simulink subsystem "massBalances"  (R2024a)
settings: Solver=VariableStepAuto  StartTime=0.0  StopTime=10.0  RelTol=1e-3
settings Model: DefaultTestHarness=massBalances_Harness1  Creator=ilan.malkin  LastModifiedBy=eunice.duplessis

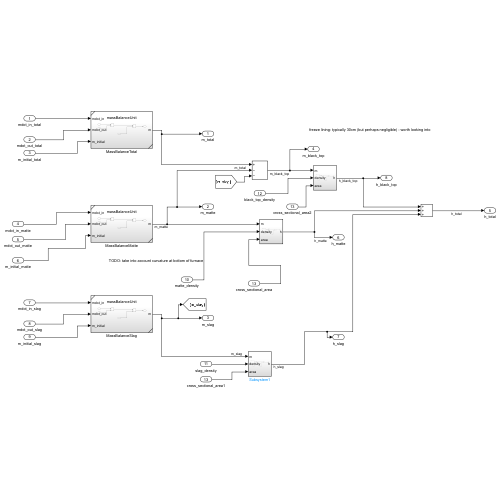
[thumbnail: Simulink's stored preview of the top-level diagram]
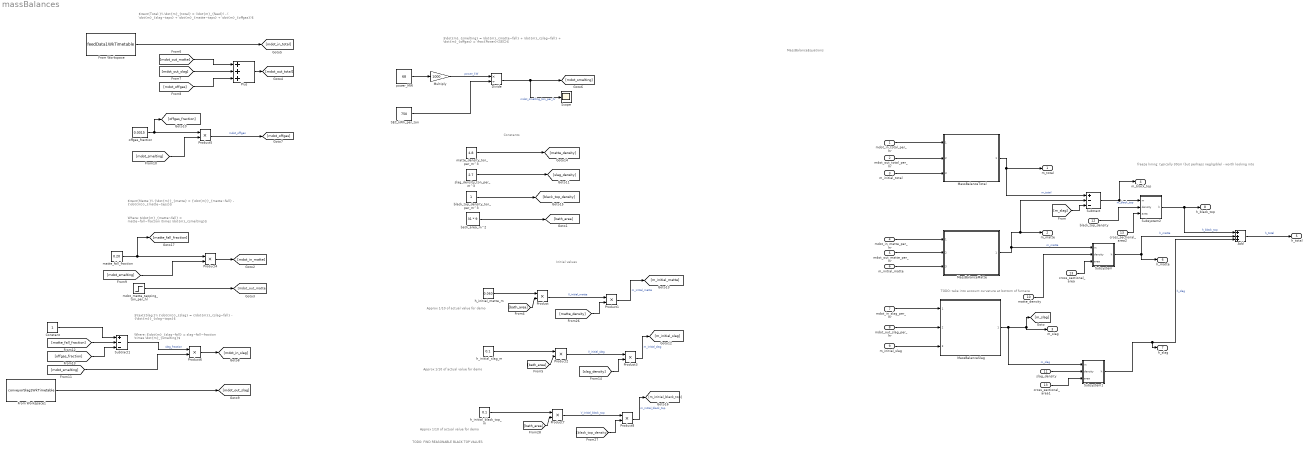
== system massBalances ==
  note: MassBalanceEquations
  note: freeze lining: typically 30cm (but perhaps negligible) - worth looking into
  note: TODO: take into account curvature at bottom of furnace
  note: $\text{Total:}\\ \dot{m}_{total} = (\dot{m}_{feed}) - ( \dot{m}_{slag~taps} + \dot{m}_{matte~taps} + \dot{m}_{offgas})$
  note: Approx 1/10 of actual value for demo
  note: $\text{Matte:}\\ {\dot{m}}_{matte} = {\dot{m}}_{matte~fall} - {\dot{m}}_{matte~taps}$
  note: Constants
  note: Initial values
  note: Approx 1/10 of actual value for demo
  note: Approx 1/10 of actual value for demo
  note: TODO: FIND REASONABLE BLACK TOP VALUES
  note: Where: $\dot{m}_{matte~fall} = matte~fall~fraction \times \dot{m}_{smelting}$
  note: Where: $\dot{m}_{slag~fall} = slag~fall~fraction \times \dot{m}_{smelting}$
  note: $\text{Slag:}\\ {\dot{m}}_{slag} = {\dot{m}}_{slag~fall} - {\dot{m}}_{slag~taps}$
  note: $\dot{m}_{smelting} = \dot{m}_{matte~fall} + \dot{m}_{slag~fall} + \dot{m}_{offgas} = \frac{Power}{SEC}$
  mdot_in_total_per_hr : Inport
  mdot_out_total_per_hr : Inport  Port=2
  m_initial_total : Inport  Port=3
  mdot_in_matte_per_hr : Inport  Port=4
  mdot_out_matte_per_hr : Inport  Port=5
  m_initial_matte : Inport  Port=6
  mdot_in_slag_per_hr : Inport  Port=7
  mdot_out_slag_per_hr : Inport  Port=8
  m_initial_slag : Inport  Port=9
  matte_density : Inport  Port=10
  slag_density : Inport  Port=11
  black_top_density : Inport  Port=12
  cross_sectional_area : Inport  Port=13
  Add : Sum  Inputs=+++
  Constant : Constant
  Divide : Product  Inputs=*/
  From Workspace : FromWorkspace  VariableName=feedData1WkTimetable
  From Workspace1 : FromWorkspace  VariableName=conveyorSlag1WkTimetable
  MassBalanceMatte : Subsystem  ReferencedSubsystem=massBalanceUnit
  MassBalanceSlag : Subsystem  ReferencedSubsystem=massBalanceUnit
  MassBalanceTotal : Subsystem  ReferencedSubsystem=massBalanceUnit
  Multiply : Gain  Gain=1000
  Plus : Sum  Inputs=+++
  Product{,1..8} (9 alike) : Product
  SEC_kWh_per_ton : Constant  Value=750
  Scope : Scope
  Subsystem : Subsystem
  Subsystem1 : Subsystem
  Subsystem2 : Subsystem
  Subtract : Sum  Inputs=+--
  Subtract1 : Sum  Inputs=+--
  bath_area_m^2 : Constant  Value=31 * 9
  black_top_density_ton_per_m^3 : Constant
  cross_sectional_area1 : InportShadow  Port=13
  cross_sectional_area2 : InportShadow  Port=13
  h_initial_black_top_m : Constant  Value=0.1
  h_initial_matte_m : Constant  Value=0.060
  h_initial_slag_m : Constant  Value=0.1
  matte_density_ton_per_m^3 : Constant  Value=4.8
  matte_fall_fraction : Constant  Value=0.20
  mdot_matte_tapping_ton_per_hr : Step  Time=44  After=1.5  SampleTime=0
  offgas_fraction : Constant  Value=0.0015
  power_MW : Constant  Value=68
  slag_density_ton_per_m^3 : Constant  Value=2.7
  m_total : Outport
  m_matte : Outport  Port=2
  m_slag : Outport  Port=3
  m_black_top : Outport  Port=4
  h_total : Outport  Port=5
  h_matte : Outport  Port=6
  h_slag : Outport  Port=7
  h_black_top : Outport  Port=8
  wires:
  MassBalanceMatte/1 -> Subsystem/1(m), Subtract/2, m_matte/1  "m_matte"
  mdot_in_matte_per_hr/1 -> MassBalanceMatte/1
  mdot_out_matte_per_hr/1 -> MassBalanceMatte/2
  m_initial_matte/1 -> MassBalanceMatte/3
  mdot_in_total_per_hr/1 -> MassBalanceTotal/1
  mdot_out_total_per_hr/1 -> MassBalanceTotal/2
  m_initial_total/1 -> MassBalanceTotal/3
  MassBalanceTotal/1 -> Subtract/1, m_total/1  "m_total"
  matte_density/1 -> Subsystem/2(density)
  cross_sectional_area/1 -> Subsystem/3(area)
  Subsystem/1(h) -> h_matte/1, Add/2  "h_matte"
  slag_density/1 -> Subsystem1/2(density)
  cross_sectional_area1/1 -> Subsystem1/3(area)
  Subsystem1/1(h) -> Add/3, h_slag/1  "h_slag"
  Add/1 -> h_total/1  "h_total"
  MassBalanceSlag/1 -> [m_slag], m_slag/1, Subsystem1/1(m)  "m_slag"
  m_initial_slag/1 -> MassBalanceSlag/3
  mdot_out_slag_per_hr/1 -> MassBalanceSlag/2
  mdot_in_slag_per_hr/1 -> MassBalanceSlag/1
  [m_slag] -> Subtract/3
  Subtract/1 -> m_black_top/1, Subsystem2/1(m)  "m_black_top"
  cross_sectional_area2/1 -> Subsystem2/3(area)
  black_top_density/1 -> Subsystem2/2(density)
  Subsystem2/1(h) -> Add/1, h_black_top/1  "h_black_top"
  mdot_matte_tapping_ton_per_hr/1 -> [mdot_out_matte]
  Product/1 -> Product1/1  "V_initial_matte"
  slag_density_ton_per_m^3/1 -> [slag_density]
  Product1/1 -> [m_initial_matte]  "m_initial_matte"
  [black_top_density] -> Product8/2
  Product7/1 -> Product8/1  "V_initial_black_top"
  Product2/1 -> Product3/1  "V_initial_slag"
  Multiply/1 -> Divide/1  "power_kW"
  offgas_fraction/1 -> Product5/1, [offgas_fraction]
  matte_fall_fraction/1 -> Product4/1, [matte_fall_fraction]
  [bath_area] -> Product2/2
  Constant/1 -> Subtract1/1
  SEC_kWh_per_ton/1 -> Divide/2
  [mdot_out_matte] -> Plus/1
  [mdot_offgas] -> Plus/3
  Subtract1/1 -> Product6/1  "slag_fraction"
  Product6/1 -> [mdot_in_slag]
  [bath_area] -> Product/2
  Product3/1 -> [m_initial_slag]  "m_initial_slag"
  [offgas_fraction] -> Subtract1/3
  matte_density_ton_per_m^3/1 -> [matte_density]
  Divide/1 -> [mdot_smelting], Scope/1  "mdot_smelting_ton_per_hr"
  Plus/1 -> [mdot_out_total]
  [mdot_smelting] -> Product6/2
  [mdot_smelting] -> Product5/2
  power_MW/1 -> Multiply/1
  black_top_density_ton_per_m^3/1 -> [black_top_density]
  [slag_density] -> Product3/2
  From Workspace/1 -> [mdot_in_total]
  [matte_fall_fraction] -> Subtract1/2
  h_initial_matte_m/1 -> Product/1
  From Workspace1/1 -> [mdot_out_slag]
  [mdot_out_slag] -> Plus/2
  Product8/1 -> [m_initial_black_top]  "m_initial_black_top"
  bath_area_m^2/1 -> [bath_area]
  [bath_area] -> Product7/2
  Product4/1 -> [mdot_in_matte]
  Product5/1 -> [mdot_offgas]  "mdot_offgas"
  h_initial_black_top_m/1 -> Product7/1
  [matte_density] -> Product1/2
  [mdot_smelting] -> Product4/2
  h_initial_slag_m/1 -> Product2/1

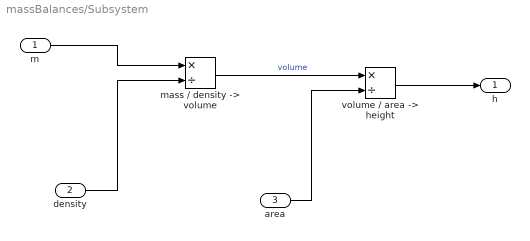
== system massBalances/Subsystem ==
  m : Inport
  density : Inport  Port=2
  area : Inport  Port=3
  "mass / density -> volume" : Product  Inputs=*/
  "volume / area -> height" : Product  Inputs=*/
  h : Outport
  wires:
  "mass / density -> volume"/1 -> "volume / area -> height"/1  "volume"
  density/1 -> "mass / density -> volume"/2
  "volume / area -> height"/1 -> h/1
  m/1 -> "mass / density -> volume"/1
  area/1 -> "volume / area -> height"/2

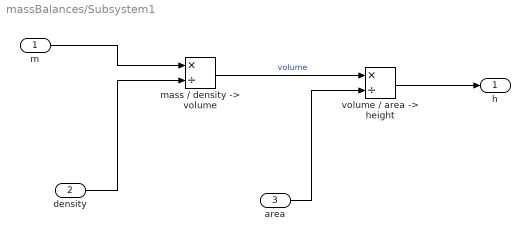
== system massBalances/Subsystem1 ==
  m : Inport
  density : Inport  Port=2
  area : Inport  Port=3
  "mass / density -> volume" : Product  Inputs=*/
  "volume / area -> height" : Product  Inputs=*/
  h : Outport
  wires:
  area/1 -> "volume / area -> height"/2
  m/1 -> "mass / density -> volume"/1
  "volume / area -> height"/1 -> h/1
  density/1 -> "mass / density -> volume"/2
  "mass / density -> volume"/1 -> "volume / area -> height"/1  "volume"

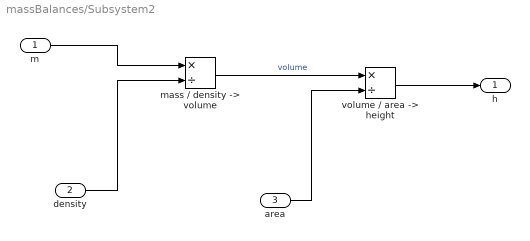
== system massBalances/Subsystem2 ==
  m : Inport
  density : Inport  Port=2
  area : Inport  Port=3
  "mass / density -> volume" : Product  Inputs=*/
  "volume / area -> height" : Product  Inputs=*/
  h : Outport
  wires:
  area/1 -> "volume / area -> height"/2
  m/1 -> "mass / density -> volume"/1
  "volume / area -> height"/1 -> h/1
  density/1 -> "mass / density -> volume"/2
  "mass / density -> volume"/1 -> "volume / area -> height"/1  "volume"
